simulink model "exam1_sim"  (R2023a)
settings: Solver=VariableStepAuto  StartTime=0.0  StopTime=10.0  RelTol=1e-9  AbsTol=1e-9
values from neighbouring files (symbols this model uses):
  r = 0.03    [exam2.m]
undefined symbols (not defined in the file or in its folder): a_0, a_1, a_2
settings Model: Creator=laptop  LastModifiedBy=laptop

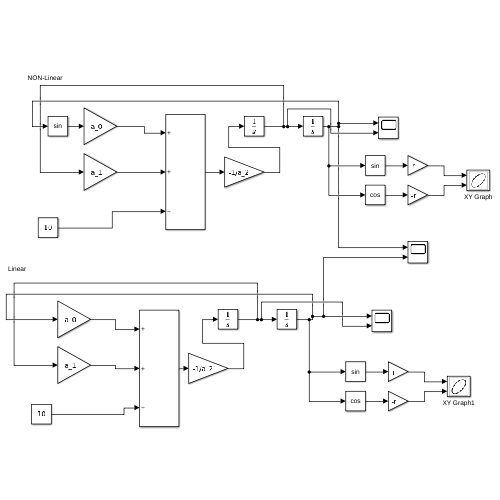
[thumbnail: Simulink's stored preview of the top-level diagram]
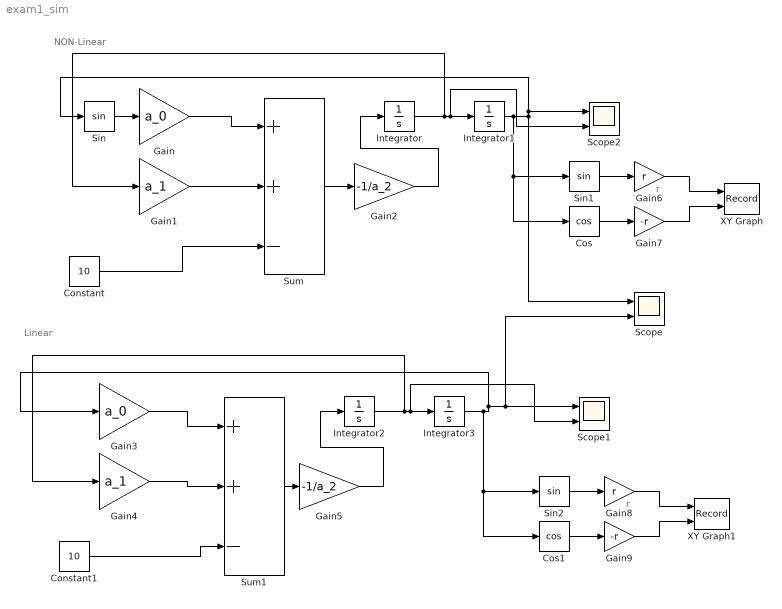
== system exam1_sim ==
  note: Linear
  note: r
  note: r
  note: NON-Linear
  Constant : Constant  Value=10
  Constant1 : Constant  Value=10
  Cos : Trigonometry  Operator=cos
  Cos1 : Trigonometry  Operator=cos
  Gain : Gain  Gain=a_0
  Gain1 : Gain  Gain=a_1
  Gain2 : Gain  Gain=-1/a_2
  Gain3 : Gain  Gain=a_0
  Gain4 : Gain  Gain=a_1
  Gain5 : Gain  Gain=-1/a_2
  Gain6 : Gain  Gain=r
  Gain7 : Gain  Gain=-r
  Gain8 : Gain  Gain=r
  Gain9 : Gain  Gain=-r
  Integrator : Integrator
  Integrator1 : Integrator  InitialCondition=pi/2
  Integrator2 : Integrator
  Integrator3 : Integrator  InitialCondition=pi/2
  Scope : Scope  NumInputPorts=2
  Scope1 : Scope  NumInputPorts=2
  Scope2 : Scope  NumInputPorts=2
  Sin : Trigonometry
  Sin1 : Trigonometry
  Sin2 : Trigonometry
  Sum : Sum  Inputs=++-
  Sum1 : Sum  Inputs=++-
  XY Graph : Record  FileSettingsInternal="{\"entries\":[{\"content\":{\"excelSettings\":{\"content\":{},\"type\":\"Streamout.ExcelSettings\"}},\"type\":\"Streamout.FileSettingStorage\",\"uuid\":\"\"}],\"packageUris\":[\"http:\\/\\/schema.mathworks.com\\/mf0\\/streamout_blocks\\/R2020a\"],\"version\":\"1.0\"}"  Layout=[1 1]  SignalsInternal="{\"entries\":[{\"content\":{\"signals\":[{\"content\":{\"blockPath\":[],\"dimensions\":[1],\"domain\":\"\",\"lineColor\":\"#a2142f\",\"plots\":[1],\"port\":1,\"sid\":[\"\"],\"signalID\":522,\"signalName\":\"Gain6\"},\"type\":\"RecordBlkView.Signal\",\"uuid\":\"\"},{\"content\":{\"blockPath\":[],\"dimensions\":[1],\"domain\":\"\",\"lineColor\":\"#139fff\",\"plots\":[1],\"port\":2,\"sid\":[\"\"],\"signalID\":526,\"signalName\":\"Gain7\"},\"type\":\"RecordBlkView.Signal\",\"uuid\":\"\"}]},\"type\":\"RecordBlkView.InputSignals\",\"uuid\":\"\"}],\"packageUris\":[\"http:\\/\\/schema.mathworks.com\\/mf0\\/streamout_blocks\\/R2020a\"],\"version\":\"1.0\"}"  VisualizationBindings="{\"xyplotplugin\":{\"info\":[{\"series\":[{\"bindingParametersList\":[{\"parameter\":\"X-Axis\",\"signalID\":522,\"signalName\":\"Gain6\"},{\"parameter\":\"Y-Axis\",\"signalID\":526,\"signalName\":\"Gain7\"}],\"seriesID\":28020}],\"subplotID\":1}]}}"  CompatibilityTag=XY
  XY Graph1 : Record  FileSettingsInternal="{\"entries\":[{\"content\":{\"excelSettings\":{\"content\":{},\"type\":\"Streamout.ExcelSettings\"}},\"type\":\"Streamout.FileSettingStorage\",\"uuid\":\"\"}],\"packageUris\":[\"http:\\/\\/schema.mathworks.com\\/mf0\\/streamout_blocks\\/R2020a\"],\"version\":\"1.0\"}"  Layout=[1 1]  SignalsInternal="{\"entries\":[{\"content\":{\"signals\":[{\"content\":{\"blockPath\":[],\"dimensions\":[1],\"domain\":\"\",\"lineColor\":\"#a2142f\",\"plots\":[1],\"port\":1,\"sid\":[\"\"],\"signalID\":530,\"signalName\":\"Gain8\"},\"type\":\"RecordBlkView.Signal\",\"uuid\":\"\"},{\"content\":{\"blockPath\":[],\"dimensions\":[1],\"domain\":\"\",\"lineColor\":\"#139fff\",\"plots\":[1],\"port\":2,\"sid\":[\"\"],\"signalID\":534,\"signalName\":\"Gain9\"},\"type\":\"RecordBlkView.Signal\",\"uuid\":\"\"}]},\"type\":\"RecordBlkView.InputSignals\",\"uuid\":\"\"}],\"packageUris\":[\"http:\\/\\/schema.mathworks.com\\/mf0\\/streamout_blocks\\/R2020a\"],\"version\":\"1.0\"}"  VisualizationBindings="{\"xyplotplugin\":{\"info\":[{\"series\":[{\"bindingParametersList\":[{\"parameter\":\"X-Axis\",\"signalID\":530,\"signalName\":\"Gain8\"},{\"parameter\":\"Y-Axis\",\"signalID\":534,\"signalName\":\"Gain9\"}],\"seriesID\":15721}],\"subplotID\":1}]}}"  CompatibilityTag=XY
  wires:
  Integrator/1 -> Gain1/1, Scope2/2, Integrator1/1
  Integrator1/1 -> Scope/1, Scope2/1, Sin/1, Cos/1, Sin1/1
  Sin/1 -> Gain/1
  Gain/1 -> Sum/1
  Gain1/1 -> Sum/2
  Gain4/1 -> Sum1/2
  Integrator2/1 -> Gain4/1, Scope1/2, Integrator3/1
  Gain3/1 -> Sum1/1
  Sin1/1 -> Gain6/1
  Cos/1 -> Gain7/1
  Gain6/1 -> XY Graph/1
  Gain7/1 -> XY Graph/2
  Integrator3/1 -> Cos1/1, Sin2/1, Scope/2, Scope1/1, Gain3/1
  Sin2/1 -> Gain8/1
  Gain9/1 -> XY Graph1/2
  Cos1/1 -> Gain9/1
  Gain8/1 -> XY Graph1/1
  Sum/1 -> Gain2/1
  Gain2/1 -> Integrator/1
  Sum1/1 -> Gain5/1
  Gain5/1 -> Integrator2/1
  Constant1/1 -> Sum1/3
  Constant/1 -> Sum/3
